simulink model "Conledspies"  (R2020b)
settings: Solver=VariableStepAuto  StartTime=0.0  StopTime=500  RelTol=1e-3
libraries: arduino_io_lib x7
settings Model: Creator=Daniel  LastModifiedBy=Daniel

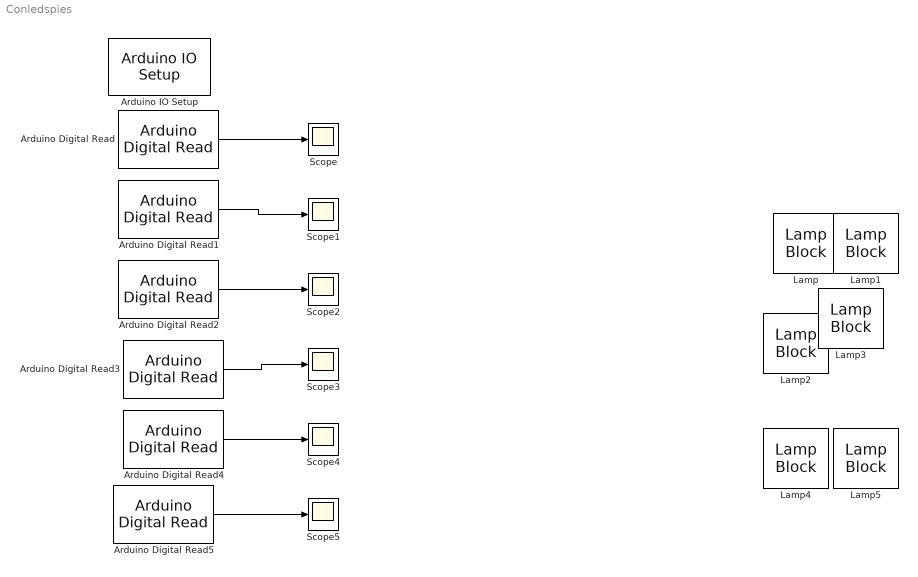
== system Conledspies ==
  Arduino Digital Read : arduino_io_lib/Arduino Digital Read  arduinoVar=Temporary arduino variable: Arduino1  arduinoPin=8  T=0.2
  Arduino Digital Read1 : arduino_io_lib/Arduino Digital Read  arduinoVar=Temporary arduino variable: Arduino1  arduinoPin=9  T=0.2
  Arduino Digital Read2 : arduino_io_lib/Arduino Digital Read  arduinoVar=Temporary arduino variable: Arduino1  arduinoPin=10  T=0.2
  Arduino Digital Read3 : arduino_io_lib/Arduino Digital Read  arduinoVar=Temporary arduino variable: Arduino1  arduinoPin=11  T=0.2
  Arduino Digital Read4 : arduino_io_lib/Arduino Digital Read  arduinoVar=Temporary arduino variable: Arduino1  arduinoPin=12  T=0.2
  Arduino Digital Read5 : arduino_io_lib/Arduino Digital Read  arduinoVar=Temporary arduino variable: Arduino1  arduinoPin=13  T=0.2
  Arduino IO Setup : arduino_io_lib/Arduino IO Setup  Priority=3  arduinoVar=Temporary arduino variable: Arduino1  workspaceVarName=a  comPort=COM4
  Lamp{,1..5} (6 alike) : LampBlock
  Scope{,1..5} (6 alike) : Scope
  wires:
  Arduino Digital Read4/1 -> Scope4/1
  Arduino Digital Read3/1 -> Scope3/1
  Arduino Digital Read2/1 -> Scope2/1
  Arduino Digital Read1/1 -> Scope1/1
  Arduino Digital Read/1 -> Scope/1
  Arduino Digital Read5/1 -> Scope5/1
